simulink model "BehCookLine"  (R2026a)
settings: Solver=VariableStepAuto
model workspace (MAT data in the model file):
  CookRate_bph = 90
  CookTau_s = 180
  PowerFull_kW = 50
  PowerIdle_kW = 8
settings Model: DataDictionary=BehParamsCommon.sldd  ParameterArgumentNames=CookRate_bph,PowerFull_kW,PowerIdle_kW,CookTau_s  Creator=sarah  LastModifiedBy=sdagen

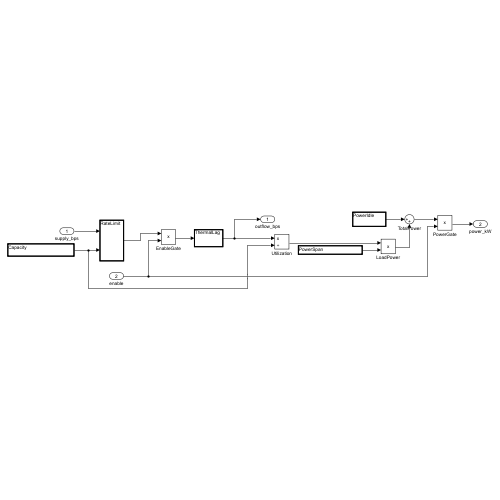
[thumbnail: Simulink's stored preview of the top-level diagram]
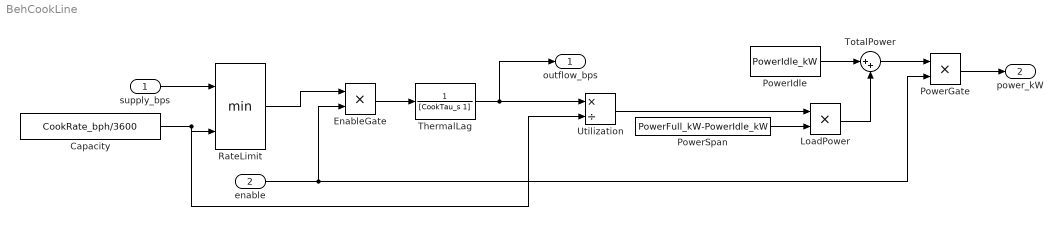
== system BehCookLine ==
  supply_bps : Inport
  enable : Inport  Port=2
  Capacity : Constant  Value=CookRate_bph/3600
  EnableGate : Product
  LoadPower : Product
  PowerGate : Product
  PowerIdle : Constant  Value=PowerIdle_kW
  PowerSpan : Constant  Value=PowerFull_kW-PowerIdle_kW
  RateLimit : MinMax  Inputs=2
  ThermalLag : TransferFcn  Denominator=[CookTau_s 1]
  TotalPower : Sum  Inputs=|++
  Utilization : Product  Inputs=*/
  outflow_bps : Outport
  power_kW : Outport  Port=2
  wires:
  supply_bps/1 -> RateLimit/1
  ThermalLag/1 -> outflow_bps/1, Utilization/1
  Capacity/1 -> Utilization/2, RateLimit/2
  RateLimit/1 -> EnableGate/1
  PowerSpan/1 -> LoadPower/2
  enable/1 -> EnableGate/2, PowerGate/2
  Utilization/1 -> LoadPower/1
  EnableGate/1 -> ThermalLag/1
  PowerIdle/1 -> TotalPower/1
  LoadPower/1 -> TotalPower/2
  TotalPower/1 -> PowerGate/1
  PowerGate/1 -> power_kW/1
